simulink model "My_SPWM"  (R2021a)
settings: Solver=ode4  StartTime=0.0  StopTime=10.0  FixedStep=1e-5  RelTol=1e-3
libraries: simulink x1, spspowerguiLib x1
settings Model: Creator=tanmoyera  LastModifiedBy=tanmoyera

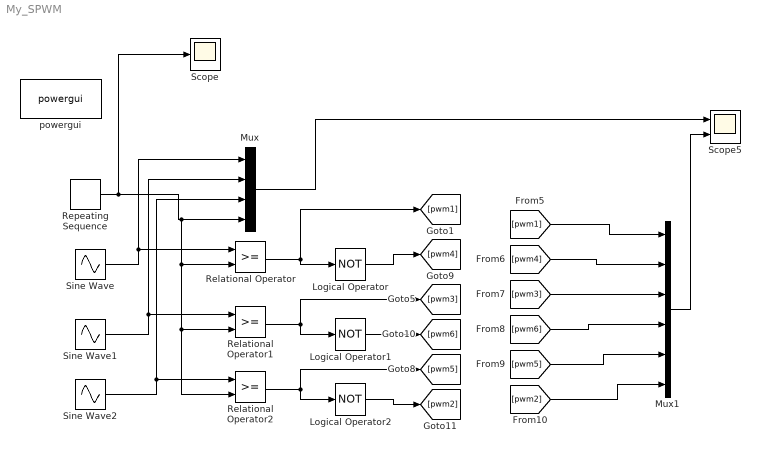
== system My_SPWM ==
  Logical Operator : Logic  Operator=NOT  AllPortsSameDT=off  OutDataTypeStr=boolean
  Logical Operator1 : Logic  Operator=NOT  AllPortsSameDT=off  OutDataTypeStr=boolean
  Logical Operator2 : Logic  Operator=NOT  AllPortsSameDT=off  OutDataTypeStr=boolean
  Mux : Mux
  Mux1 : Mux  Inputs=6
  Relational Operator : RelationalOperator  OutDataTypeStr=boolean  RndMeth=Simplest
  Relational Operator1 : RelationalOperator  OutDataTypeStr=boolean  RndMeth=Simplest
  Relational Operator2 : RelationalOperator  OutDataTypeStr=boolean  RndMeth=Simplest
  Repeating Sequence : simulink/Sources/Repeating Sequence  rep_seq_t=[0 1 2 3]*[1/6000]  rep_seq_y=[0 1 -1 0]
  Scope : Scope
  Scope5 : Scope  NumInputPorts=2
  Sine Wave : Sin  Frequency=2*pi*50  SampleTime=0
  Sine Wave1 : Sin  Frequency=2*pi*50  Phase=2*pi/3  SampleTime=0
  Sine Wave2 : Sin  Frequency=2*pi*50  Phase=-2*pi/3  SampleTime=0
  powergui : spspowerguiLib/powergui  Priority=1  SimulationMode=Continuous  SampleTime=50e-6  frequency=60  Iterations=50  frequencyindice=60  Pbase=100e6  ErrMax=1e-4  UnitsV=kV  UnitsW=MW  buscounter=0  FunctionMessages=off  echomessages=off  EnableUseOfTLC=off  CurrentSourceSwitches=off  DisableSnubberDevices=off  DisableRonSwitches=off  DisableVfSwitches=off  DisplayEquations=off  AutomaticDiscreteSolvers=off  SolverType=Tustin/Backward Euler (TBE)  Interpol=off  ExternalGateDelay=off  methode=off  Ts=100  x0status=blocks  SPID=on  SwTol=0  HookPort=off  NonlinearTolerance=1e-4  nMaxIteration=100  ContinueOnMaxIteration=off  RestoreLinks=warning  ResistiveCurrentMeasurement=off  Frange=[0:2:500]  Ylog=off  Xlog=on  ShowGrid=off  save=off  variable=ZData  structure=0  ZoomFFT=off  StartTime=0.0  cycles=1  DisplayStyle=1  fundamental=60  FreqAxis=off  MaxFrequency=1000  frequencyindicesteady=1  RmsSteady=1  display=off
  wires:
  [pwm2] -> Mux1/6
  Mux/1 -> Scope5/1
  Relational Operator/1 -> Logical Operator/1, [pwm1]
  Sine Wave/1 -> Relational Operator/1, Mux/1
  Logical Operator2/1 -> [pwm2]
  Logical Operator/1 -> [pwm4]
  Repeating Sequence/1 -> Scope/1, Relational Operator/2, Relational Operator1/2, Relational Operator2/2, Mux/4
  Sine Wave1/1 -> Relational Operator1/1, Mux/2
  Relational Operator1/1 -> [pwm3], Logical Operator1/1
  [pwm6] -> Mux1/4
  [pwm5] -> Mux1/5
  [pwm1] -> Mux1/1
  Logical Operator1/1 -> [pwm6]
  Relational Operator2/1 -> [pwm5], Logical Operator2/1
  [pwm4] -> Mux1/2
  Sine Wave2/1 -> Relational Operator2/1, Mux/3
  [pwm3] -> Mux1/3
  Mux1/1 -> Scope5/2
